simulink model "Iridium18"  (R2018a)
settings: Solver=FixedStepAuto  StartTime=0.0  StopTime=2*3600  FixedStep=dt  RelTol=1e-3
values from neighbouring files (symbols this model uses):
  a = -mu/(2*xi)    [AA279A_ECI2OE.m]    (also in AA279A_HW2.m = rp/(1-e(ii)); ECI2OE.m = inf; Halleys_Comet_Call.m = 2667966400; ISS_Call.m = 6781.5)
  e = norm(e_vec)    [AA279A_ECI2OE.m]    (also in AA279A_HW2.m = [0.7 0.0 1.9 1.0]; ECI2OE.m = norm(eVec); Halleys_Comet_Call.m = 0.967; ISS_Call.m = 0.0006483)
  i = acosd(h(3)/hnorm)    [AA279A_ECI2OE.m]    (also in ECI2OE.m = acosd(hVec(3)/h); ISS_Call.m = 0.901326422973; Iridium18_Call.m = 1.50785975397; Molniya331_Call.m = deg2rad(i))
  InitialDate = [2018, 4, 22]    [ISS_Call.m]    (also in Iridium18_Call.m = 57421.510593; Molniya331_Call.m = [2018, 2, 1])
  lambda_GS = -122.173355*(pi/180)    (= -2.13232730296)    [Iridium18_Call.m]
  M0 = 0    [Halleys_Comet_Call.m]    (also in ISS_Call.m = 0.9101; Iridium18_Call.m = 0.475253155318; Molniya331_Call.m = E - e*sin(E))
  n = [-h(2);h(1);0]    [AA279A_ECI2OE.m]    (also in AA279A_OE2ECI.m = sqrt(mu/a^3); ECI2OE.m = norm(nVec); Halleys_Comet_Call.m = sqrt(mu/(a^3)); ISS_Call.m = sqrt(mu/(a^3)))
  phi_GS = 37.426622*(pi/180)    (= 0.653217781799)    [Iridium18_Call.m]
  RAAN = RAAN + 360    [AA279A_ECI2OE.m]    (also in ISS_Call.m = 1.41506932429; Iridium18_Call.m = 4.02952891054; Molniya331_Call.m = deg2rad(RAAN))
  w = 360 - w    [AA279A_ECI2OE.m]    (also in ECI2OE.m; ISS_Call.m = 0.685300040137; Iridium18_Call.m = 1.56927789035; Molniya331_Call.m = deg2rad(w))
settings Model: Creator=Marquito  LastModifiedBy=Marquito

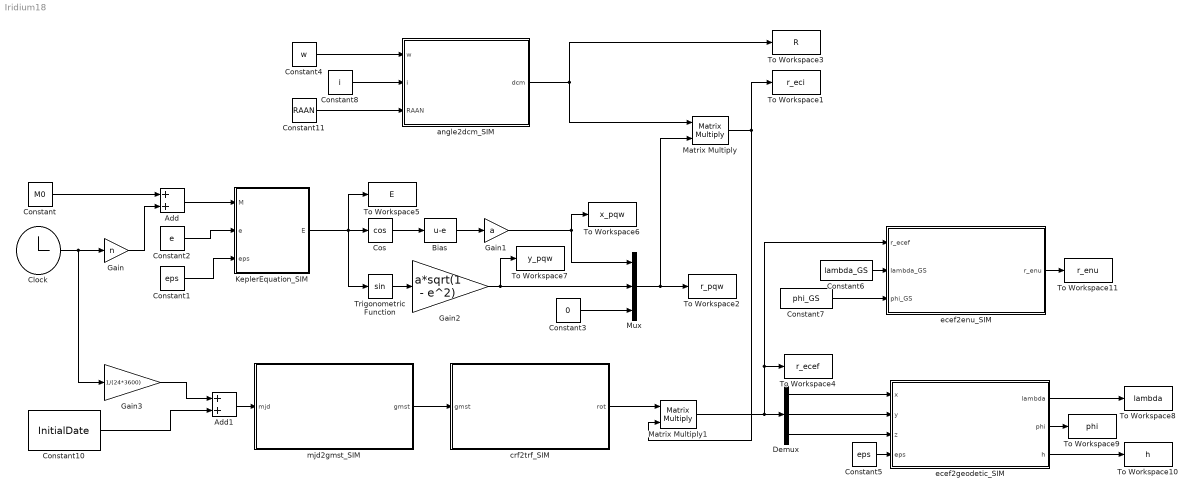
== system Iridium18 ==
  Add : Sum
  Add1 : Sum
  Bias : Bias  Bias=-e
  Clock : Clock
  Constant : Constant  Value=M0
  Constant1 : Constant  Value=eps
  Constant10 : Constant  Value=InitialDate
  Constant11 : Constant  Value=RAAN
  Constant2 : Constant  Value=e
  Constant3 : Constant  Value=0
  Constant4 : Constant  Value=w
  Constant5 : Constant  Value=eps
  Constant6 : Constant  Value=lambda_GS
  Constant7 : Constant  Value=phi_GS
  Constant8 : Constant  Value=i
  Cos : Trigonometry  Operator=cos
  Demux : Demux  Outputs=3
  Gain : Gain  Gain=n
  Gain1 : Gain  Gain=a
  Gain2 : Gain  Gain=a*sqrt(1 - e^2)
  Gain3 : Gain  Gain=1/(24*3600)
  KeplerEquation_SIM : MATLAB Function  TreatAsAtomicUnit=on
  Matrix Multiply : Product  Multiplication=Matrix(*)
  Matrix Multiply1 : Product  Multiplication=Matrix(*)
  Mux : Mux  Inputs=3
  To Workspace1 : ToWorkspace  VariableName=r_eci  SampleTime=-1
  To Workspace10 : ToWorkspace  VariableName=h  SampleTime=-1
  To Workspace11 : ToWorkspace  VariableName=r_enu  SampleTime=-1
  To Workspace2 : ToWorkspace  VariableName=r_pqw  SampleTime=-1
  To Workspace3 : ToWorkspace  VariableName=R  SampleTime=-1
  To Workspace4 : ToWorkspace  VariableName=r_ecef  SampleTime=-1
  To Workspace5 : ToWorkspace  VariableName=E  SampleTime=-1
  To Workspace6 : ToWorkspace  VariableName=x_pqw  SampleTime=-1
  To Workspace7 : ToWorkspace  VariableName=y_pqw  SampleTime=-1
  To Workspace8 : ToWorkspace  VariableName=lambda  SampleTime=-1
  To Workspace9 : ToWorkspace  VariableName=phi  SampleTime=-1
  Trigonometric Function : Trigonometry
  angle2dcm_SIM : MATLAB Function  TreatAsAtomicUnit=on
  crf2trf_SIM : MATLAB Function  TreatAsAtomicUnit=on
  ecef2enu_SIM : MATLAB Function  TreatAsAtomicUnit=on
  ecef2geodetic_SIM : MATLAB Function  TreatAsAtomicUnit=on
  mjd2gmst_SIM : MATLAB Function  TreatAsAtomicUnit=on
  wires:
  Add/1 -> KeplerEquation_SIM/1(M)
  KeplerEquation_SIM/1(E) -> Trigonometric Function/1, To Workspace5/1, Cos/1
  Constant2/1 -> KeplerEquation_SIM/2(e)
  Constant1/1 -> KeplerEquation_SIM/3(eps)
  angle2dcm_SIM/1(dcm) -> To Workspace3/1, Matrix Multiply/1
  mjd2gmst_SIM/1(gmst) -> crf2trf_SIM/1(gmst)
  crf2trf_SIM/1(rot) -> Matrix Multiply1/1
  Matrix Multiply1/1 -> To Workspace4/1, ecef2enu_SIM/1(r_ecef), Demux/1
  Constant/1 -> Add/1
  Gain/1 -> Add/2
  Cos/1 -> Bias/1
  Bias/1 -> Gain1/1
  Gain1/1 -> To Workspace6/1, Mux/1
  Trigonometric Function/1 -> Gain2/1
  Gain2/1 -> To Workspace7/1, Mux/2
  Constant3/1 -> Mux/3
  Mux/1 -> To Workspace2/1, Matrix Multiply/2
  Matrix Multiply/1 -> To Workspace1/1, Matrix Multiply1/2
  Constant8/1 -> angle2dcm_SIM/2(i)
  Constant11/1 -> angle2dcm_SIM/3(RAAN)
  Constant4/1 -> angle2dcm_SIM/1(w)
  Clock/1 -> Gain3/1, Gain/1
  Demux/1 -> ecef2geodetic_SIM/1(x)
  Demux/2 -> ecef2geodetic_SIM/2(y)
  Demux/3 -> ecef2geodetic_SIM/3(z)
  Constant5/1 -> ecef2geodetic_SIM/4(eps)
  ecef2geodetic_SIM/3(h) -> To Workspace10/1
  ecef2geodetic_SIM/2(phi) -> To Workspace9/1
  ecef2geodetic_SIM/1(lambda) -> To Workspace8/1
  Add1/1 -> mjd2gmst_SIM/1(mjd)
  Constant10/1 -> Add1/2
  Gain3/1 -> Add1/1
  Constant6/1 -> ecef2enu_SIM/2(lambda_GS)
  Constant7/1 -> ecef2enu_SIM/3(phi_GS)
  ecef2enu_SIM/1(r_enu) -> To Workspace11/1

== matlab function Iridium18/ecef2geodetic_SIM ==
  data: x input; lambda output; y input; z input; eps input; phi output; h output
function [lambda, phi, h] = ecef2geodetic(x, y, z, eps)
% ecef2geod Converts ECEF coordinates to Geodetic latitude and longitude
%
% Inputs :
% x - ECEF x coordinate [km]
% y - ECEF y coordinate [km]
% z - ECEF z coordinate [km]
% eps - tolerance of coordinate result [deg]
%
% Outputs :
% lambda - Geodetic longitude of orbit [deg]
% phi - Geodetic latitude of orbit [deg]
% h - Geodetic altitude of orbit [km]

rE = 6378.1; % Earth Equatorial Radius 
eE = 0.0818; % WGS84 Ellipsoid Eccentricity

r = sqrt(x.^2 + y.^2 + z.^2);
lambda = atan2d(y, x); % Geocentric Longitude = Geodetic Longitude

phi_i = asin(z./r); % Use geocentric latitude as first guess
N = rE/sqrt(1 - eE^2*(sin(phi_i)^2)); % Modified Radius of Curvature
r_xy = sqrt(x.^2 + y.^2);
diff = 2*eps;

while abs(diff) > eps
    phi1 = atan2d((z + N*eE^2*sin(phi_i)), r_xy);
    diff = phi1 - phi_i;
    phi_i = phi1;
    N = rE/sqrt(1 - eE^2*(sin(phi_i)^2));
end

phi = phi_i;
h = r_xy/cosd(phi) - N;

end

== matlab function Iridium18/KeplerEquation_SIM ==
  data: M input; E output; e input; eps input
function E = KeplerEq(M,e,eps)
% Function solves Kepler's equation M = E-e*sin(E)
% Input - Mean Anomaly M [rad], Eccentricity e, and Epsilon 
% Output - Eccentric anomaly E [rad] 
M = mod(M, 2*pi);
En  = M;
Ens = En - (En-e*sin(En)- M)/(1 - e*cos(En));
while ( abs(Ens-En) > eps )
	En = Ens;
	Ens = En - (En - e*sin(En) - M)/(1 - e*cos(En));
end
E = Ens;
end

== matlab function Iridium18/mjd2gmst_SIM ==
  data: mjd input; gmst output
function gmst = mjd2gmst(mjd)
% mjd2gmst  Converts  UT1 time in MJD to GMST in  radians
%
% Inputs:
%    mjd   - Modified  Julian  Date  Value [d]
%
% Outputs:
%    gmst - Greenwich  Mean  Sidereal  Time [rad]

d = mjd - 51544.5; % Normalize  by  epoch (Jan. 1, 2000  12:00h)

gmst_deg = 280.4606 + 360.9856473*d;
gmst_rad = pi/180*gmst_deg;

gmst = mod(gmst_rad, 2*pi);

end

== matlab function Iridium18/angle2dcm_SIM ==
  data: w input; i input; dcm output; RAAN input
function dcm  = angle2dcm(w, i, RAAN)
% dcm = angle2dcm(r1,r2,r3,seq)
% builds euler angle rotation matrix
% 
% r = [r1 r2 r3]
% seq = 'ZYX' (default)
%       'ZXZ'
% dcm = direction cosine matrix

dcm = eye(3,3);
r = [-w; -i; -RAAN];
seq = 'ZXZ';

switch seq
  case 'ZYX'
    dcm = Tx(r(3))*Ty(r(2))*Tz(r(1));
  case 'ZXZ'
    dcm = Tz(r(3))*Tx(r(2))*Tz(r(1)); 
end

function A = Tx(a)
A = [1 0 0;
    0 cos(a) sin(a);
    0 -sin(a) cos(a)];
end

function A = Ty(a)
A = [cos(a) 0 -sin(a);
    0 1 0;
    sin(a) 0 cos(a)];
end

function A = Tz(a)
A = [cos(a) sin(a) 0;
    -sin(a) cos(a) 0;
    0 0 1];
end

end

== matlab function Iridium18/crf2trf_SIM ==
  data: gmst input; rot output
function rot = crf2trf(gmst)
% crf2trf  Creates a rotation  matrix  between  CRF  and  TRFsystems
%
% Inputs:
%    gmst - Greenwich  Mean  Sidereal  Time [rad]
%
% Outputs:
%    rot   - rotation  matrix  from  celestial  to  terrestrial reference  
%            frames

rot = rotz(-gmst);

end

== matlab function Iridium18/ecef2enu_SIM ==
  data: r_ecef input; lambda_GS input; r_enu output; phi_GS input
function r_enu = ecef2enu(r_ecef, lambda_GS, phi_GS)
% ecef2enu Converts ECEF position to ENU position
%
% Note : This function assumes an elliptical Earth
%
% Inputs :
% lam_gs - Ground station Geodetic longitude [ rad ]
% phi_gs - Ground station Geodetic latitude [ rad ]
% r_ecef - Satellite ECEF position vector [km]
%
% Outputs :
% r_enu - Satellite ENU position vector [km]

% Earth parameters
r_E = 6378.1;
e_E = 0.0818;

% Compute the satellite position wrt the ground station in ECEF
N = r_E/sqrt(1 - e_E^2*(sin(phi_GS)^2));
r_GS_ecef = [N*cos(phi_GS)*cos(lambda_GS);
            N*cos(phi_GS)*sin(lambda_GS);
            N*(1 - e_E)*sin(phi_GS)];
r_sat_GS = r_ecef - r_GS_ecef;

% Develop the ECEF to ENU rotation matrix
E = [-sin(lambda_GS);
    cos(lambda_GS);
    0];
N = [-sin(phi_GS)*cos(lambda_GS);
    -sin(phi_GS)*sin(lambda_GS);
    cos(phi_GS)];
U = [cos(phi_GS)*cos(lambda_GS);
    cos(phi_GS)*sin(lambda_GS);
    sin(phi_GS)];

Recef2enu = [E, N, U]';

% Rotate the position vector into ENU coordinates
r_enu = Recef2enu*r_sat_GS;

end
